simulink model "ex4"  (R2023a)
settings: Solver=VariableStepAuto  StartTime=0.0  StopTime=t_sim+5  FixedStep=1e-3  RelTol=1e-3
values from neighbouring files (symbols this model uses):
  b = 0.2    [ex3_4.m]
  k1 = 5    [ex3_4.m]    (also in ex5.m = 1)
  k2 = 5    [ex3_4.m]    (also in ex5.m = 2.5)
  qi = [0; 0; 0]    [ex3_4.m]
libraries: robotmobilelib x1
settings Model: Creator=Francesco  LastModifiedBy=salvatoregranata
settings OptimizationCC: ReuseModelBlockBuffer=off

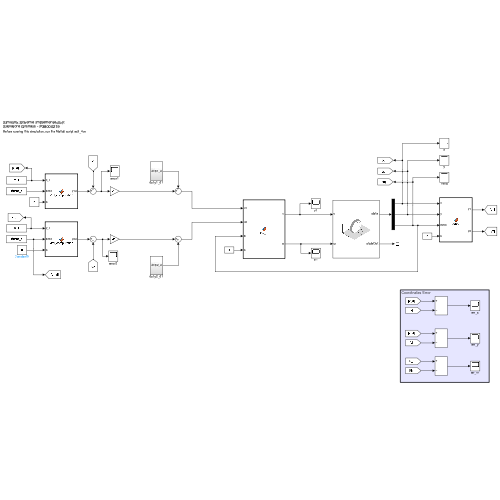
[thumbnail: Simulink's stored preview of the top-level diagram]
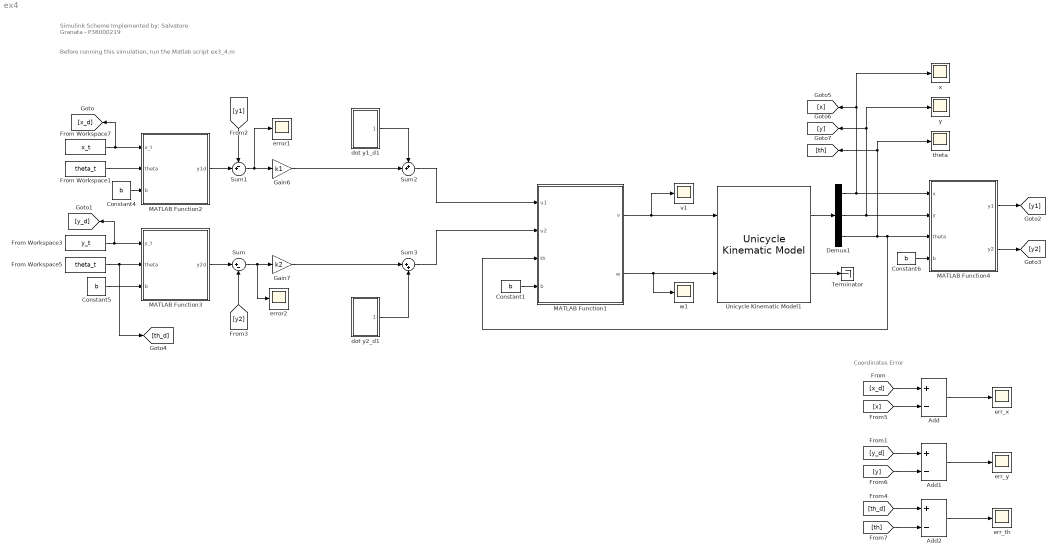
== system ex4 ==
  note: Coordinates Error
  note: Before running this simulation, run the Matlab script ex3_4.m
  note: Simulink Scheme Implemented by:
      | Salvatore Granata - P38000219
  Add : Sum  Inputs=+-
  Add1 : Sum  Inputs=+-
  Add2 : Sum  Inputs=+-
  Constant{1,4..6} (4 alike) : Constant  Value=b
  Demux1 : Demux  Outputs=3
  From Workspace1 : FromWorkspace  VariableName=theta_t  OutputAfterFinalValue=Holding final value
  From Workspace3 : FromWorkspace  VariableName=y_t  OutputAfterFinalValue=Holding final value
  From Workspace5 : FromWorkspace  VariableName=theta_t  OutputAfterFinalValue=Holding final value
  From Workspace7 : FromWorkspace  VariableName=x_t  OutputAfterFinalValue=Holding final value
  Gain6 : Gain  Gain=k1
  Gain7 : Gain  Gain=k2
  MATLAB Function1 : MATLAB Function  TreatAsAtomicUnit=on
  MATLAB Function2 : MATLAB Function  TreatAsAtomicUnit=on
  MATLAB Function3 : MATLAB Function  TreatAsAtomicUnit=on
  MATLAB Function4 : MATLAB Function  TreatAsAtomicUnit=on
  Sum : Sum  Inputs=|+-
  Sum1 : Sum  Inputs=-+|
  Sum2 : Sum  Inputs=++|
  Sum3 : Sum  Inputs=|++
  Terminator : Terminator
  Unicycle Kinematic Model1 : robotmobilelib/Unicycle Kinematic Model  VehicleInputs=Vehicle Speed & Heading Angular Velocity  WheelRadius=0.1  WheelSpeedRange=[-Inf Inf]  InitialState=[qi]  SimulateUsing=Interpreted execution
  dot y1_d1 : Subsystem
  dot y2_d1 : Subsystem
  err_th : Scope
  err_x : Scope
  err_y : Scope
  error1 : Scope
  error2 : Scope
  theta : Scope
  v1 : Scope
  w1 : Scope
  x : Scope
  y : Scope
  wires:
  Unicycle Kinematic Model1/1 -> Demux1/1
  MATLAB Function1/1(v) -> Unicycle Kinematic Model1/1, v1/1
  [y1] -> Sum1/1
  Sum/1 -> Gain7/1, error2/1
  [y2] -> Sum/2
  Sum1/1 -> Gain6/1, error1/1
  Demux1/3 -> MATLAB Function4/3(theta), MATLAB Function1/3(th), [th], theta/1
  Sum2/1 -> MATLAB Function1/1(u1)
  Constant1/1 -> MATLAB Function1/4(b)
  MATLAB Function1/2(w) -> Unicycle Kinematic Model1/2, w1/1
  Demux1/1 -> MATLAB Function4/1(x), [x], x/1
  Constant5/1 -> MATLAB Function3/3(b)
  From Workspace5/1 -> [th_d], MATLAB Function3/2(theta)
  Demux1/2 -> MATLAB Function4/2(y), [y], y/1
  Sum3/1 -> MATLAB Function1/2(u2)
  From Workspace7/1 -> MATLAB Function2/1(x_t), [x_d]
  From Workspace1/1 -> MATLAB Function2/2(theta)
  Constant4/1 -> MATLAB Function2/3(b)
  MATLAB Function2/1(y1d) -> Sum1/2
  From Workspace3/1 -> [y_d], MATLAB Function3/1(y_t)
  MATLAB Function3/1(y2d) -> Sum/1
  Constant6/1 -> MATLAB Function4/4(b)
  MATLAB Function4/1(y1) -> [y1]
  MATLAB Function4/2(y2) -> [y2]
  dot y1_d1/1(doty1_d) -> Sum2/1
  Gain6/1 -> Sum2/2
  Gain7/1 -> Sum3/1
  dot y2_d1/1(doty2_d) -> Sum3/2
  Add2/1 -> err_th/1
  Add1/1 -> err_y/1
  Add/1 -> err_x/1
  [x_d] -> Add/1
  [y_d] -> Add1/1
  [th_d] -> Add2/1
  [x] -> Add/2
  [y] -> Add1/2
  [th] -> Add2/2
  Unicycle Kinematic Model1/2 -> Terminator/1

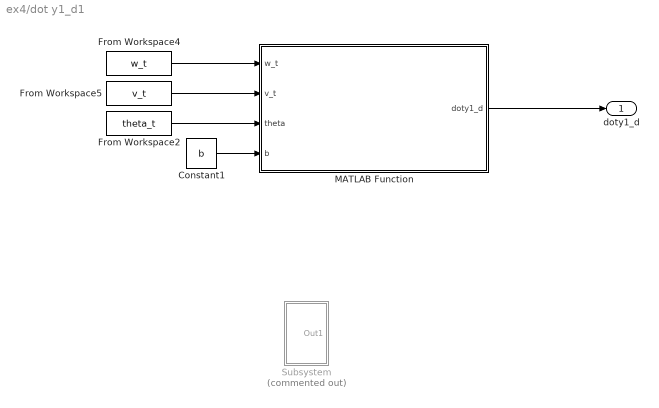
== system ex4/dot y1_d1 ==
  Constant1 : Constant  Value=b
  From Workspace2 : FromWorkspace  VariableName=theta_t  OutputAfterFinalValue=Holding final value
  From Workspace4 : FromWorkspace  VariableName=w_t  OutputAfterFinalValue=Holding final value
  From Workspace5 : FromWorkspace  VariableName=v_t  OutputAfterFinalValue=Holding final value
  MATLAB Function : MATLAB Function  TreatAsAtomicUnit=on
  Subsystem : Subsystem  Commented=on
  doty1_d : Outport
  wires:
  From Workspace2/1 -> MATLAB Function/3(theta)
  From Workspace4/1 -> MATLAB Function/1(w_t)
  Constant1/1 -> MATLAB Function/4(b)
  From Workspace5/1 -> MATLAB Function/2(v_t)
  MATLAB Function/1(doty1_d) -> doty1_d/1

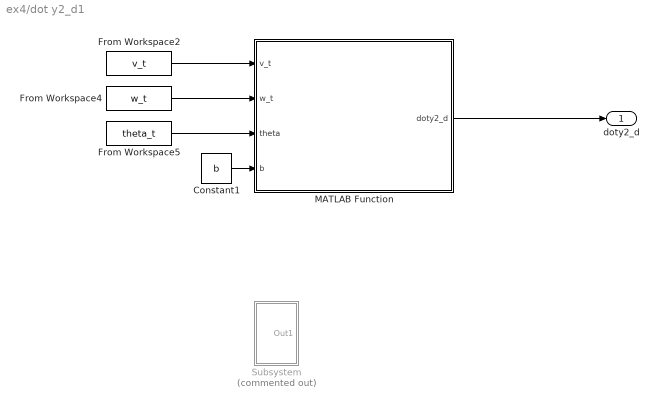
== system ex4/dot y2_d1 ==
  Constant1 : Constant  Value=b
  From Workspace2 : FromWorkspace  VariableName=v_t  OutputAfterFinalValue=Holding final value
  From Workspace4 : FromWorkspace  VariableName=w_t  OutputAfterFinalValue=Holding final value
  From Workspace5 : FromWorkspace  VariableName=theta_t  OutputAfterFinalValue=Holding final value
  MATLAB Function : MATLAB Function  TreatAsAtomicUnit=on
  Subsystem : Subsystem  Commented=on
  doty2_d : Outport
  wires:
  From Workspace2/1 -> MATLAB Function/1(v_t)
  From Workspace4/1 -> MATLAB Function/2(w_t)
  From Workspace5/1 -> MATLAB Function/3(theta)
  Constant1/1 -> MATLAB Function/4(b)
  MATLAB Function/1(doty2_d) -> doty2_d/1

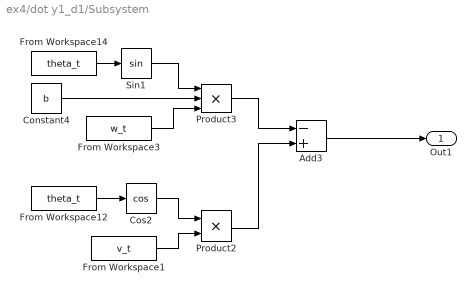
== system ex4/dot y1_d1/Subsystem ==
  Add3 : Sum  Inputs=-+
  Constant4 : Constant  Value=b
  Cos2 : Trigonometry  Operator=cos
  From Workspace1 : FromWorkspace  VariableName=v_t  OutputAfterFinalValue=Holding final value
  From Workspace12 : FromWorkspace  VariableName=theta_t  OutputAfterFinalValue=Holding final value
  From Workspace14 : FromWorkspace  VariableName=theta_t  OutputAfterFinalValue=Holding final value
  From Workspace3 : FromWorkspace  VariableName=w_t  OutputAfterFinalValue=Holding final value
  Product2 : Product
  Product3 : Product  Inputs=3
  Sin1 : Trigonometry
  Out1 : Outport
  wires:
  From Workspace12/1 -> Cos2/1
  From Workspace14/1 -> Sin1/1
  From Workspace3/1 -> Product3/3
  Constant4/1 -> Product3/2
  Cos2/1 -> Product2/1
  Add3/1 -> Out1/1
  Product2/1 -> Add3/2
  Product3/1 -> Add3/1
  From Workspace1/1 -> Product2/2
  Sin1/1 -> Product3/1

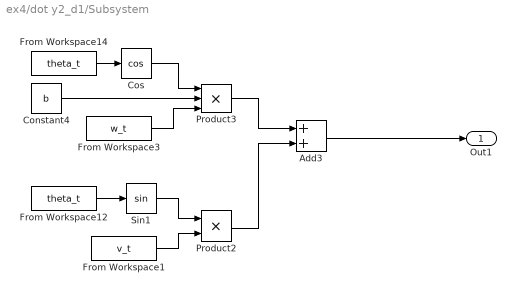
== system ex4/dot y2_d1/Subsystem ==
  Add3 : Sum
  Constant4 : Constant  Value=b
  Cos : Trigonometry  Operator=cos
  From Workspace1 : FromWorkspace  VariableName=v_t  OutputAfterFinalValue=Holding final value
  From Workspace12 : FromWorkspace  VariableName=theta_t  OutputAfterFinalValue=Holding final value
  From Workspace14 : FromWorkspace  VariableName=theta_t  OutputAfterFinalValue=Holding final value
  From Workspace3 : FromWorkspace  VariableName=w_t  OutputAfterFinalValue=Holding final value
  Product2 : Product
  Product3 : Product  Inputs=3
  Sin1 : Trigonometry
  Out1 : Outport
  wires:
  Constant4/1 -> Product3/2
  Cos/1 -> Product3/1
  Sin1/1 -> Product2/1
  Add3/1 -> Out1/1
  From Workspace12/1 -> Sin1/1
  From Workspace14/1 -> Cos/1
  From Workspace3/1 -> Product3/3
  From Workspace1/1 -> Product2/2
  Product3/1 -> Add3/1
  Product2/1 -> Add3/2

== matlab function ex4/MATLAB Function1 ==
  data: u1 input; v output; u2 input; th input; w output; b input
function [v,w] = inv_T(u1,u2,th,b)
     v=u1*cos(th)+u2*sin(th);
     w=-u1*sin(th)/b+u2*cos(th)/b;

== matlab function ex4/MATLAB Function2 ==
  data: x_t input; theta input; y1d output; b input
function y1d = y1d_computation(x_t,theta,b)
    
y1d = x_t+b*cos(theta);

== matlab function ex4/dot y1_d1/MATLAB Function ==
  data: w_t input; v_t input; doty1_d output; theta input; b input
function doty1_d = dot_y1d_computation(w_t, v_t ,theta,b)

doty1_d = v_t*cos(theta) - w_t*b*sin(theta);

== matlab function ex4/MATLAB Function3 ==
  data: y_t input; theta input; y2d output; b input
function y2d = y2d_computation(y_t,theta,b)
    
y2d = y_t+b*sin(theta);

== matlab function ex4/dot y2_d1/MATLAB Function ==
  data: v_t input; doty2_d output; w_t input; theta input; b input
function doty2_d = doty2_d_computation(v_t,w_t,theta,b)

doty2_d=v_t*sin(theta)+w_t*b*cos(theta)

== matlab function ex4/MATLAB Function4 ==
  data: x input; y1 output; y input; theta input; y2 output; b input
function [y1,y2] = output(x,y,theta,b)
y1=x+b*cos(theta);
y2=y+b*sin(theta);
